simulink model "P1_Part1"  (R2023b)
settings: Solver=ode1  StartTime=0.0  StopTime=25  FixedStep=dT  RelTol=1e-3
values from neighbouring files (symbols this model uses):
  A = 1    [P1_Week2_Update (1).m]    (also in P1_Week2_Update.m; Project1_Part1.m)
  b = index3    [P1_Week2_Update (1).m]    (also in P1_Week2_Update.m; Project1_Part1.m)
  f = index7    [P1_Week2_Update (1).m]    (also in P1_Week2_Update.m; Project1_Part1.m)
  J = index2    [P1_Week2_Update (1).m]    (also in P1_Week2_Update.m; Project1_Part1.m)
  phi = 0    [P1_Week2_Update (1).m]    (also in P1_Week2_Update.m; Project1_Part1.m)
  w_0 = index1    [P1_Week2_Update (1).m]    (also in P1_Week2_Update.m; Project1_Part1.m)
settings Model: Creator=dxego  LastModifiedBy=luker

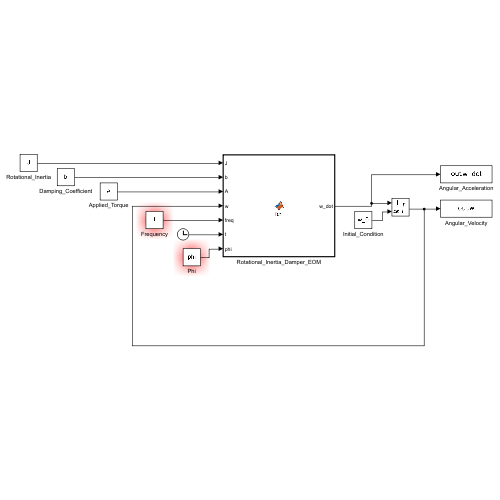
[thumbnail: Simulink's stored preview of the top-level diagram]
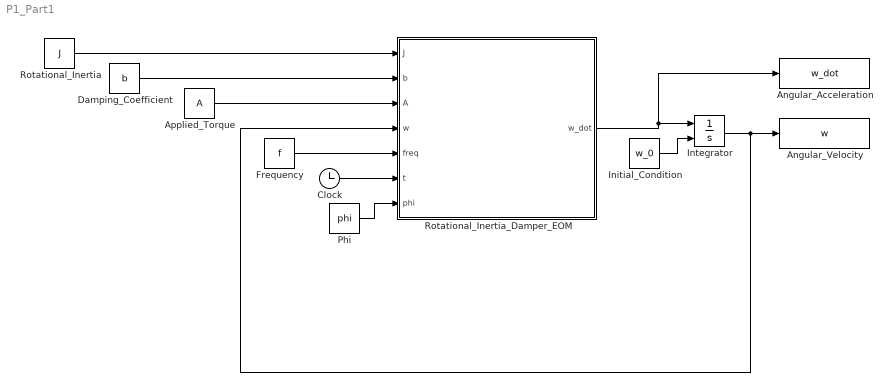
== system P1_Part1 ==
  Angular_Acceleration : ToWorkspace  VariableName=w_dot  SaveFormat=Timeseries  SampleTime=-1
  Angular_Velocity : ToWorkspace  VariableName=w  SaveFormat=Timeseries  SampleTime=-1
  Applied_Torque : Constant  Value=A
  Clock : Clock
  Damping_Coefficient : Constant  Value=b
  Frequency : Constant  Value=f
  Initial_Condition : Constant  Value=w_0
  Integrator : Integrator  InitialConditionSource=external  LimitOutput=on  UpperSaturationLimit=<binary blob, 304 chars, not shown>  LowerSaturationLimit=<binary blob, 305 chars, not shown>
  Phi : Constant  Value=phi
  Rotational_Inertia : Constant  Value=J
  Rotational_Inertia_Damper_EOM : MATLAB Function  TreatAsAtomicUnit=on
  wires:
  Rotational_Inertia/1 -> Rotational_Inertia_Damper_EOM/1(J)
  Damping_Coefficient/1 -> Rotational_Inertia_Damper_EOM/2(b)
  Applied_Torque/1 -> Rotational_Inertia_Damper_EOM/3(A)
  Rotational_Inertia_Damper_EOM/1(w_dot) -> Angular_Acceleration/1, Integrator/1
  Integrator/1 -> Rotational_Inertia_Damper_EOM/4(w), Angular_Velocity/1
  Initial_Condition/1 -> Integrator/2
  Phi/1 -> Rotational_Inertia_Damper_EOM/7(phi)
  Clock/1 -> Rotational_Inertia_Damper_EOM/6(t)
  Frequency/1 -> Rotational_Inertia_Damper_EOM/5(freq)

== matlab function P1_Part1/Rotational_Inertia_Damper_EOM ==
  data: J input; w_dot output; b input; A input; w input; freq input; t input; phi input
function w_dot = fcn(J, b, A, w, freq, t, phi)
% Recall EOM: J*w_dot = tau_applied - tau_damped
tau_damped = b*w;
tau = A*sin(freq*t+phi);
w_dot = (1/J)*(tau - tau_damped);
end
